simulink model "signal_injection"  (R2023a)
settings: Solver=FixedStepAuto  StartTime=0.0  StopTime=1/(f_fund)/6  FixedStep=1e-7  RelTol=1e-3
InitFcn:
  | f_fund=50;
  | ma=1;
  | fsw=100e3;
settings Model: Creator=enesa  LastModifiedBy=enesa

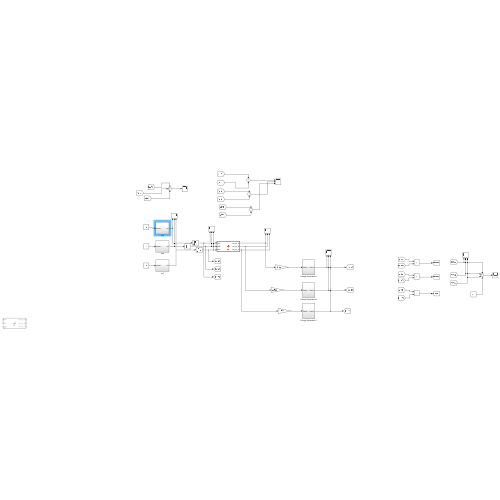
[thumbnail: Simulink's stored preview of the top-level diagram]
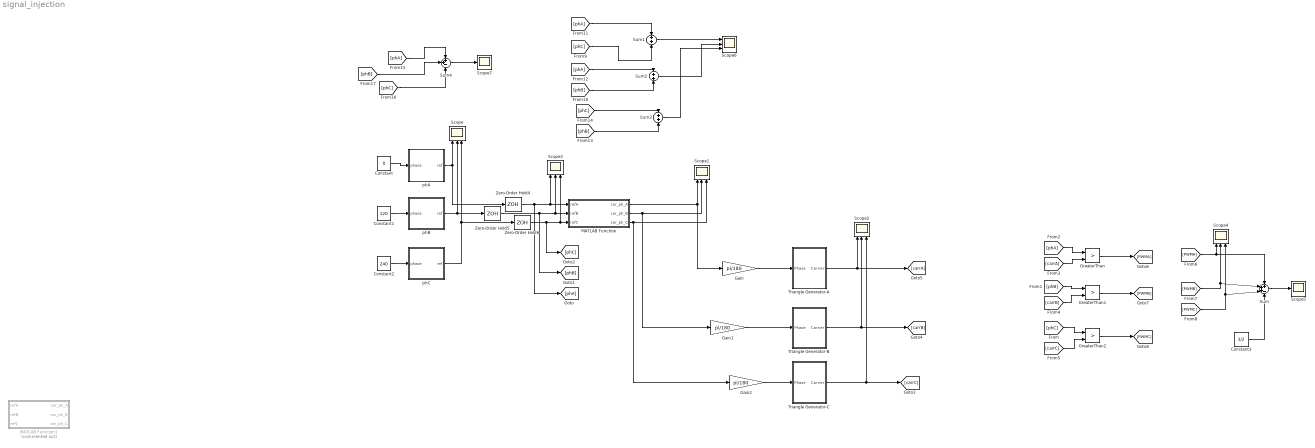
== system signal_injection ==
  Constant : Constant  Value=0
  Constant1 : Constant  Value=120
  Constant2 : Constant  Value=240
  Constant3 : Constant  Value=3/2
  Gain : Gain  Gain=pi/180
  Gain1 : Gain  Gain=pi/180
  Gain2 : Gain  Gain=pi/180
  GreaterThan : RelationalOperator  Operator=>  OutDataTypeStr=boolean  RndMeth=Simplest  InputSameDT=off
  GreaterThan1 : RelationalOperator  Operator=>  OutDataTypeStr=boolean  RndMeth=Simplest  InputSameDT=off
  GreaterThan2 : RelationalOperator  Operator=>  OutDataTypeStr=boolean  RndMeth=Simplest  InputSameDT=off
  MATLAB Function : MATLAB Function  TreatAsAtomicUnit=on
  MATLAB Function1 : MATLAB Function  Commented=on  TreatAsAtomicUnit=on
  Scope{,1..4,6} (6 alike) : Scope  NumInputPorts=3
  Scope5 : Scope
  Scope7 : Scope
  Sum : Sum  Inputs=+++-
  Sum1 : Sum
  Sum2 : Sum
  Sum3 : Sum
  Sum4 : Sum  Inputs=++-
  Triangle Generator-A : Subsystem
  Triangle Generator-B : Subsystem
  Triangle Generator-C : Subsystem
  Zero-Order Hold4 : ZeroOrderHold  SampleTime=20/fsw
  Zero-Order Hold5 : ZeroOrderHold  SampleTime=20/fsw
  Zero-Order Hold6 : ZeroOrderHold  SampleTime=20/fsw
  phA : Subsystem
  phB : Subsystem
  phC : Subsystem
  wires:
  Constant/1 -> phA/1(phase)
  Constant1/1 -> phB/1(phase)
  Constant2/1 -> phC/1(phase)
  phA/1(ref) -> Scope/1, Zero-Order Hold4/1
  phB/1(ref) -> Scope/2, Zero-Order Hold5/1
  phC/1(ref) -> Scope/3, Zero-Order Hold6/1
  MATLAB Function/1(car_ph_A) -> Gain/1, Scope1/1
  MATLAB Function/3(car_ph_C) -> Gain2/1, Scope1/3
  MATLAB Function/2(car_ph_B) -> Gain1/1, Scope1/2
  Triangle Generator-B/1(Carrier) -> [carrB], Scope2/2
  Triangle Generator-C/1(Carrier) -> [carrC], Scope2/3
  Zero-Order Hold4/1 -> Scope3/1, MATLAB Function/1(refA), [phA]
  Zero-Order Hold5/1 -> [phB], Scope3/2, MATLAB Function/2(refB)
  Zero-Order Hold6/1 -> [phC], Scope3/3, MATLAB Function/3(refC)
  Triangle Generator-A/1(Carrier) -> [carrA], Scope2/1
  [phA] -> GreaterThan/1
  [carrA] -> GreaterThan/2
  [phB] -> GreaterThan1/1
  [carrB] -> GreaterThan1/2
  [phC] -> GreaterThan2/1
  [carrC] -> GreaterThan2/2
  GreaterThan/1 -> [PWMA]
  GreaterThan1/1 -> [PWMB]
  GreaterThan2/1 -> [PWMC]
  [PWMA] -> Sum/1, Scope4/1
  [PWMB] -> Sum/2, Scope4/2
  [PWMC] -> Sum/3, Scope4/3
  Gain/1 -> Triangle Generator-A/1(Phase)
  Gain1/1 -> Triangle Generator-B/1(Phase)
  Gain2/1 -> Triangle Generator-C/1(Phase)
  Sum/1 -> Scope5/1
  Constant3/1 -> Sum/4
  [phA] -> Sum1/1
  [phC] -> Sum1/2
  Sum1/1 -> Scope6/1
  [phA] -> Sum2/1
  [phB] -> Sum2/2
  Sum2/1 -> Scope6/2
  [phB] -> Sum3/2
  [phC] -> Sum3/1
  Sum3/1 -> Scope6/3
  [phA] -> Sum4/1
  [phC] -> Sum4/3
  [phB] -> Sum4/2
  Sum4/1 -> Scope7/1

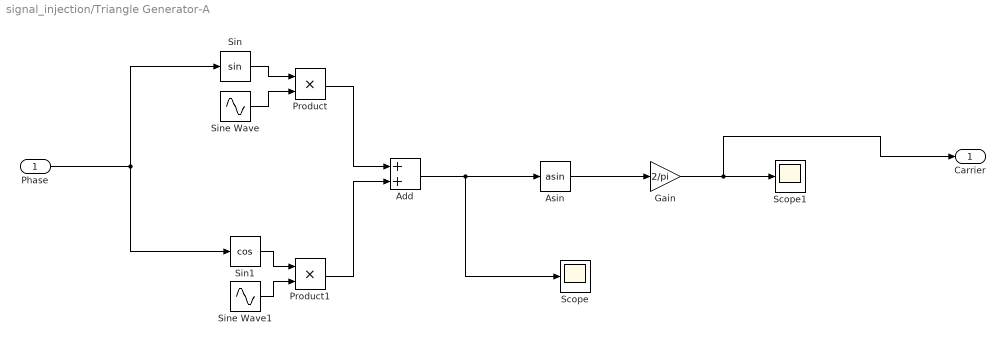
== system signal_injection/Triangle Generator-A ==
  Phase : Inport
  Add : Sum
  Asin : Trigonometry  Operator=asin
  Gain : Gain  Gain=2/pi
  Product : Product
  Product1 : Product
  Scope : Scope
  Scope1 : Scope
  Sin : Trigonometry
  Sin1 : Trigonometry  Operator=cos
  Sine Wave : Sin  Frequency=2*pi*fsw  SampleTime=0
  Sine Wave1 : Sin  Frequency=2*pi*fsw  Phase=-pi/2  SampleTime=0
  Carrier : Outport
  wires:
  Sin/1 -> Product/1
  Sine Wave/1 -> Product/2
  Phase/1 -> Sin/1, Sin1/1
  Product/1 -> Add/1
  Asin/1 -> Gain/1
  Gain/1 -> Carrier/1, Scope1/1
  Sine Wave1/1 -> Product1/2
  Product1/1 -> Add/2
  Add/1 -> Asin/1, Scope/1
  Sin1/1 -> Product1/1

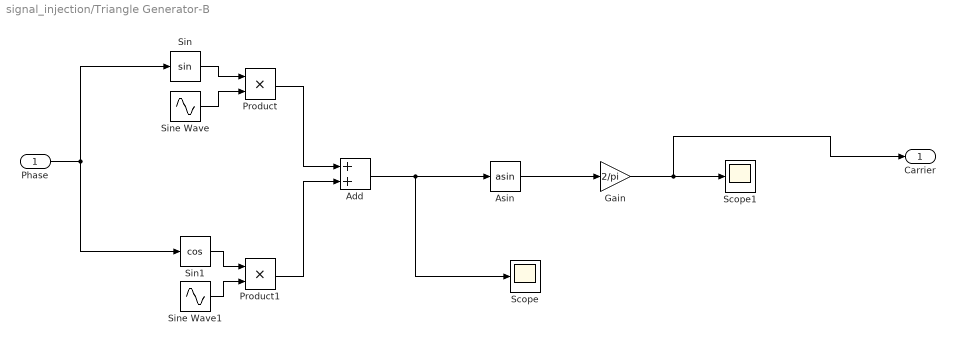
== system signal_injection/Triangle Generator-B ==
  Phase : Inport
  Add : Sum
  Asin : Trigonometry  Operator=asin
  Gain : Gain  Gain=2/pi
  Product : Product
  Product1 : Product
  Scope : Scope
  Scope1 : Scope
  Sin : Trigonometry
  Sin1 : Trigonometry  Operator=cos
  Sine Wave : Sin  Frequency=2*pi*fsw  SampleTime=0
  Sine Wave1 : Sin  Frequency=2*pi*fsw  Phase=-pi/2  SampleTime=0
  Carrier : Outport
  wires:
  Sin/1 -> Product/1
  Sine Wave/1 -> Product/2
  Phase/1 -> Sin1/1, Sin/1
  Product/1 -> Add/1
  Asin/1 -> Gain/1
  Gain/1 -> Carrier/1, Scope1/1
  Sine Wave1/1 -> Product1/2
  Product1/1 -> Add/2
  Add/1 -> Asin/1, Scope/1
  Sin1/1 -> Product1/1

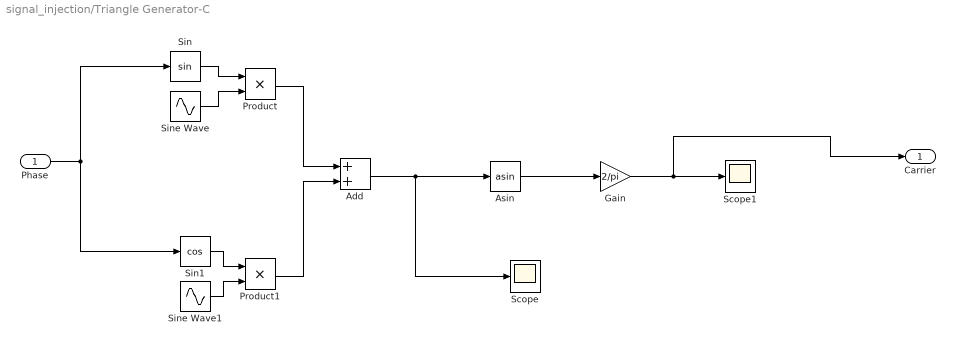
== system signal_injection/Triangle Generator-C ==
  Phase : Inport
  Add : Sum
  Asin : Trigonometry  Operator=asin
  Gain : Gain  Gain=2/pi
  Product : Product
  Product1 : Product
  Scope : Scope
  Scope1 : Scope
  Sin : Trigonometry
  Sin1 : Trigonometry  Operator=cos
  Sine Wave : Sin  Frequency=2*pi*fsw  SampleTime=0
  Sine Wave1 : Sin  Frequency=2*pi*fsw  Phase=-pi/2  SampleTime=0
  Carrier : Outport
  wires:
  Sin/1 -> Product/1
  Sine Wave/1 -> Product/2
  Phase/1 -> Sin1/1, Sin/1
  Product/1 -> Add/1
  Asin/1 -> Gain/1
  Gain/1 -> Carrier/1, Scope1/1
  Sine Wave1/1 -> Product1/2
  Product1/1 -> Add/2
  Add/1 -> Asin/1, Scope/1
  Sin1/1 -> Product1/1

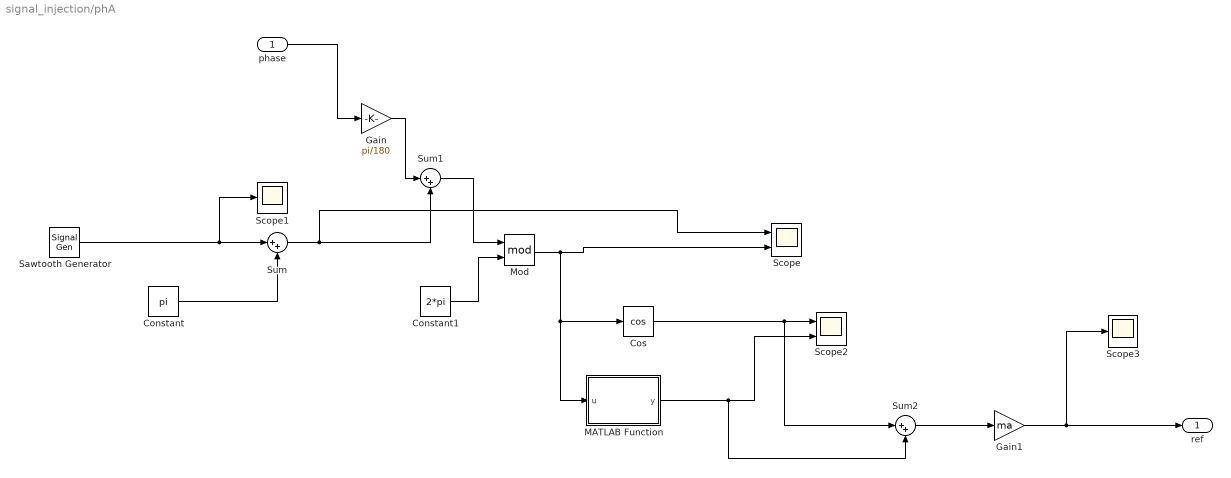
== system signal_injection/phA ==
  phase : Inport
  Constant : Constant  Value=pi
  Constant1 : Constant  Value=2*pi
  Cos : Trigonometry  Operator=cos
  Gain : Gain  Gain=pi/180
  Gain1 : Gain  Gain=ma
  MATLAB Function : MATLAB Function  TreatAsAtomicUnit=on
  Mod : Math  Operator=mod
  Sawtooth Generator : SignalGenerator  WaveForm=sawtooth  Amplitude=pi  Frequency=f_fund
  Scope : Scope  NumInputPorts=2
  Scope1 : Scope
  Scope2 : Scope  NumInputPorts=2
  Scope3 : Scope
  Sum : Sum  Inputs=|++
  Sum1 : Sum  Inputs=|++
  Sum2 : Sum  Inputs=|++
  ref : Outport
  wires:
  phase/1 -> Gain/1
  Sawtooth Generator/1 -> Scope1/1, Sum/1
  Sum/1 -> Sum1/2, Scope/1
  MATLAB Function/1(y) -> Sum2/2, Scope2/2
  Constant/1 -> Sum/2
  Mod/1 -> MATLAB Function/1(u), Cos/1, Scope/2
  Constant1/1 -> Mod/2
  Cos/1 -> Sum2/1, Scope2/1
  Sum1/1 -> Mod/1
  Sum2/1 -> Gain1/1
  Gain/1 -> Sum1/1
  Gain1/1 -> ref/1, Scope3/1

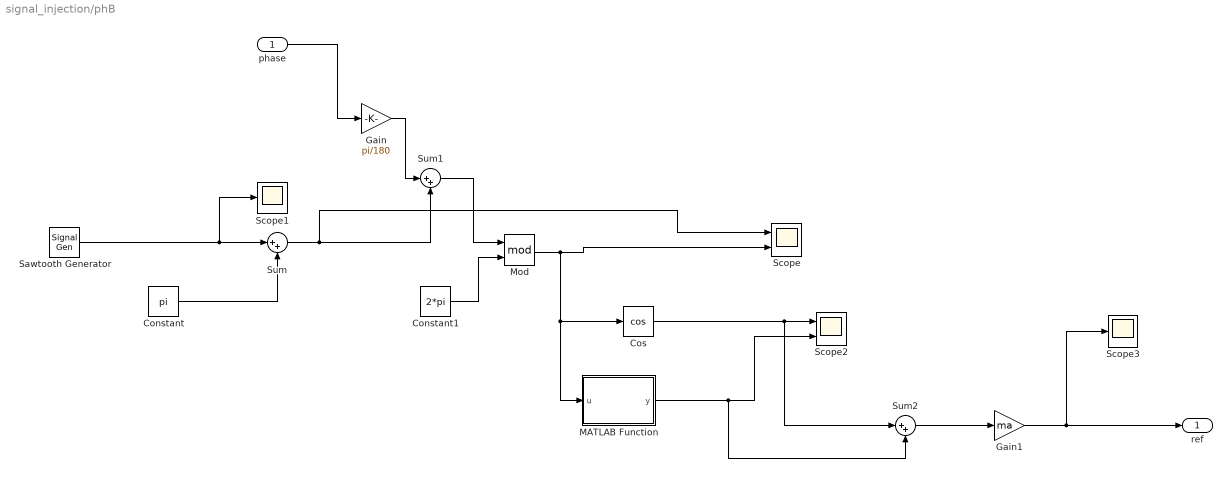
== system signal_injection/phB ==
  phase : Inport
  Constant : Constant  Value=pi
  Constant1 : Constant  Value=2*pi
  Cos : Trigonometry  Operator=cos
  Gain : Gain  Gain=pi/180
  Gain1 : Gain  Gain=ma
  MATLAB Function : MATLAB Function  TreatAsAtomicUnit=on
  Mod : Math  Operator=mod
  Sawtooth Generator : SignalGenerator  WaveForm=sawtooth  Amplitude=pi  Frequency=f_fund
  Scope : Scope  NumInputPorts=2
  Scope1 : Scope
  Scope2 : Scope  NumInputPorts=2
  Scope3 : Scope
  Sum : Sum  Inputs=|++
  Sum1 : Sum  Inputs=|++
  Sum2 : Sum  Inputs=|++
  ref : Outport
  wires:
  phase/1 -> Gain/1
  Sawtooth Generator/1 -> Scope1/1, Sum/1
  Sum/1 -> Sum1/2, Scope/1
  MATLAB Function/1(y) -> Sum2/2, Scope2/2
  Constant/1 -> Sum/2
  Mod/1 -> MATLAB Function/1(u), Cos/1, Scope/2
  Constant1/1 -> Mod/2
  Cos/1 -> Sum2/1, Scope2/1
  Sum1/1 -> Mod/1
  Sum2/1 -> Gain1/1
  Gain/1 -> Sum1/1
  Gain1/1 -> ref/1, Scope3/1

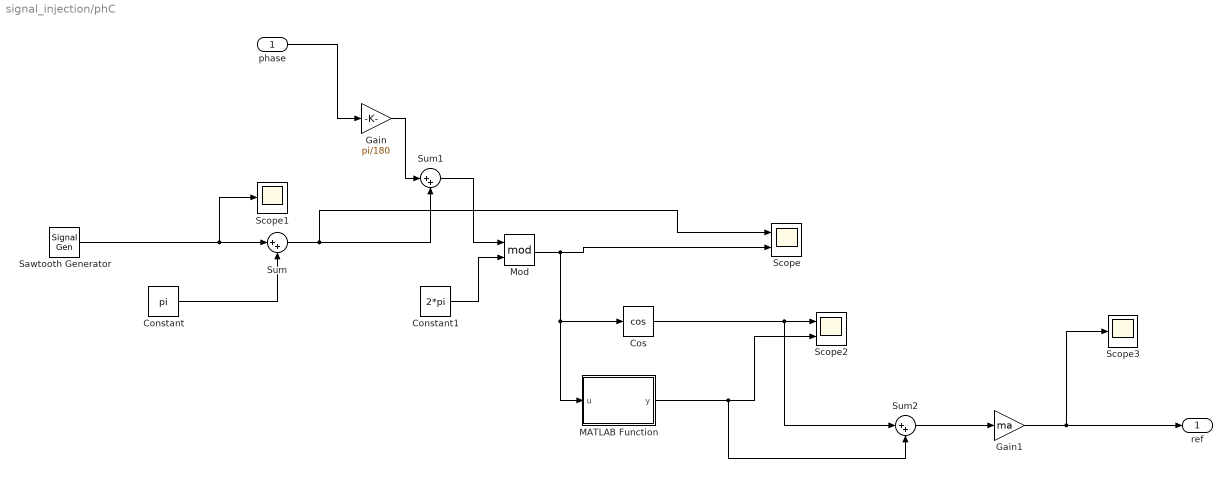
== system signal_injection/phC ==
  phase : Inport
  Constant : Constant  Value=pi
  Constant1 : Constant  Value=2*pi
  Cos : Trigonometry  Operator=cos
  Gain : Gain  Gain=pi/180
  Gain1 : Gain  Gain=ma
  MATLAB Function : MATLAB Function  TreatAsAtomicUnit=on
  Mod : Math  Operator=mod
  Sawtooth Generator : SignalGenerator  WaveForm=sawtooth  Amplitude=pi  Frequency=f_fund
  Scope : Scope  NumInputPorts=2
  Scope1 : Scope
  Scope2 : Scope  NumInputPorts=2
  Scope3 : Scope
  Sum : Sum  Inputs=|++
  Sum1 : Sum  Inputs=|++
  Sum2 : Sum  Inputs=|++
  ref : Outport
  wires:
  phase/1 -> Gain/1
  Sawtooth Generator/1 -> Scope1/1, Sum/1
  Sum/1 -> Sum1/2, Scope/1
  MATLAB Function/1(y) -> Sum2/2, Scope2/2
  Constant/1 -> Sum/2
  Mod/1 -> MATLAB Function/1(u), Cos/1, Scope/2
  Constant1/1 -> Mod/2
  Cos/1 -> Sum2/1, Scope2/1
  Sum1/1 -> Mod/1
  Sum2/1 -> Gain1/1
  Gain/1 -> Sum1/1
  Gain1/1 -> ref/1, Scope3/1

== matlab function signal_injection/phB/MATLAB Function ==
  data: u input; y output
function y = fcn(u)


if u<=2*pi && u>5*2*pi/6

    y= -(u-5*pi/3)*3/(2*pi)+1/8;

elseif u<=5*2*pi/6 && u>4*2*pi/6

    y= 0;

elseif u<=4*2*pi/6 && u>3*2*pi/6

       y= -(u-4*pi/3)*3/(2*pi)+1/8;

elseif u<=3*2*pi/6 && u>2*2*pi/6

        y= (u-2*pi/3)*3/(2*pi)+1/8;

elseif u<=2*2*pi/6 && u>1*2*pi/6

        y= 0;

elseif u<=2*pi/6 && u>=0

            y= (u-pi/3)*3/(2*pi)+1/8;

else 
    y=0;

end

== matlab function signal_injection/phA/MATLAB Function ==
  data: u input; y output
function y = fcn(u)


if u<=2*pi && u>5*2*pi/6

    y= -(u-5*pi/3)*3/(2*pi)+1/8;

elseif u<=5*2*pi/6 && u>4*2*pi/6

    y= 0;

elseif u<=4*2*pi/6 && u>3*2*pi/6

       y= -(u-4*pi/3)*3/(2*pi)+1/8;

elseif u<=3*2*pi/6 && u>2*2*pi/6

        y= (u-2*pi/3)*3/(2*pi)+1/8;

elseif u<=2*2*pi/6 && u>1*2*pi/6

        y= 0;

elseif u<=2*pi/6 && u>=0

            y= (u-pi/3)*3/(2*pi)+1/8;

else 
    y=0;

end

== matlab function signal_injection/phC/MATLAB Function ==
  data: u input; y output
function y = fcn(u)


if u<=2*pi && u>5*2*pi/6

    y= -(u-5*pi/3)*3/(2*pi)+1/8;

elseif u<=5*2*pi/6 && u>4*2*pi/6

    y= 0;

elseif u<=4*2*pi/6 && u>3*2*pi/6

       y= -(u-4*pi/3)*3/(2*pi)+1/8;

elseif u<=3*2*pi/6 && u>2*2*pi/6

        y= (u-2*pi/3)*3/(2*pi)+1/8;

elseif u<=2*2*pi/6 && u>1*2*pi/6

        y= 0;

elseif u<=2*pi/6 && u>=0

            y= (u-pi/3)*3/(2*pi)+1/8;

else 
    y=0;

end

== matlab function signal_injection/MATLAB Function ==
  data: refA input; car_ph_A output; refB input; refC input; car_ph_B output; car_ph_C output
function [car_ph_A, car_ph_B, car_ph_C]= fcn(refA, refB, refC)

refA2=(1+refA)/2;
refB2=(1+refB)/2;
refC2=(1+refC)/2,

if refA2>=refB2 && refA2>=refC2

if refB2>=refC2 
car_ph_B=0;
car_ph_C=((refA2-refC2)/2)*360;
car_ph_A=((refA2+refB2-2*refC2)/2)*360;
else
car_ph_C=0;
car_ph_B=((refA2-refB2)/2)*360;
car_ph_A=((refA2+refC2-2*refB2)/2)*360;
end

elseif refB2>=refA2 && refB2>=refC2

if refA2>=refC2 
car_ph_A=0;
car_ph_C=((refB2-refC2)/2)*360;
car_ph_B=((refA2+refB2-2*refC2)/2)*360;
else
car_ph_C=0;
car_ph_A=((refB2-refA2)/2)*360;
car_ph_B=((refB2+refC2-2*refA2)/2)*360;
end

elseif refC2>=refA2 && refC2>=refB2

if refA2>=refB2 
car_ph_A=0;
car_ph_B=((refC2-refB2)/2)*360;
car_ph_C=((refA2+refC2-2*refB2)/2)*360;

else
car_ph_B=0;
car_ph_A=((refC2-refA2)/2)*360;
car_ph_C=((refB2+refC2-2*refA2)/2)*360;

end


else

car_ph_A=0;
car_ph_B=0;
car_ph_C=0;

end





end

== matlab function signal_injection/MATLAB Function1 ==
  data: refA input; car_ph_A output; refB input; refC input; car_ph_B output; car_ph_C output
function [car_ph_A, car_ph_B, car_ph_C]= fcn(refA, refB, refC)

refA2=(1+refA)/2;
refB2=(1+refB)/2;
refC2=(1+refC)/2,

if refA2>=refB2 && refA2>=refC2

car_ph_A=0;

if refB2>=refC2 

car_ph_C=((refA2-refC2)/2)*360;
car_ph_B=((refA2+refB2-2*refC2)/2)*360;

else

car_ph_B=((refA2-refB2)/2)*360;
car_ph_C=((refA2+refC2-2*refB2)/2)*360;

end

elseif refB2>=refA2 && refB2>=refC2

car_ph_B=0;

if refA2>=refC2 

car_ph_C=((refB2-refC2)/2)*360;
car_ph_A=((refA2+refB2-2*refC2)/2)*360;

else

car_ph_A=((refB2-refA2)/2)*360;
car_ph_C=((refB2+refC2-2*refA2)/2)*360;

end

elseif refC2>=refA2 && refC2>=refB2

car_ph_C=0;

if refA2>=refB2 

car_ph_B=((refC2-refB2)/2)*360;
car_ph_A=((refA2+refC2-2*refB2)/2)*360;

else

car_ph_A=((refC2-refA2)/2)*360;
car_ph_B=((refB2+refC2-2*refA2)/2)*360;

end


else

car_ph_A=0;
car_ph_B=0;
car_ph_C=0;

end





end
